simulink model "EISGov_SelectParameter"  (R2016b)
settings: configuration reference "CodeGenConfigSet" (kept outside this file)
values from neighbouring files (symbols this model uses):
  EISGov_SetPLoRmpSlopeNeg_C = Calibration.Parameter    [init_EISGov_SelectParameter.m]    (also in init_EISGov_SelectParameter_SIL.m = Simulink.Parameter)
  EISGov_SetPLoRmpSlopePos_C = Calibration.Parameter    [init_EISGov_SelectParameter.m]    (also in init_EISGov_SelectParameter_SIL.m = Simulink.Parameter)
  EISGov_stPrio_CA = Calibration.Parameter    [init_EISGov_SelectParameter.m]    (also in init_EISGov_SelectParameter_SIL.m = Simulink.Parameter)
undefined symbols (not defined in the file or in its folder): EISGov_num_conv, EISGov_SelectParameter_DT, Switch_conv
libraries: simulink x20, CXLib x3
(part 1 of 2)
settings Model: Creator=lenovo  LastModifiedBy=xuxingpei
settings ConfigSetRef: SourceLocation=Base Workspace

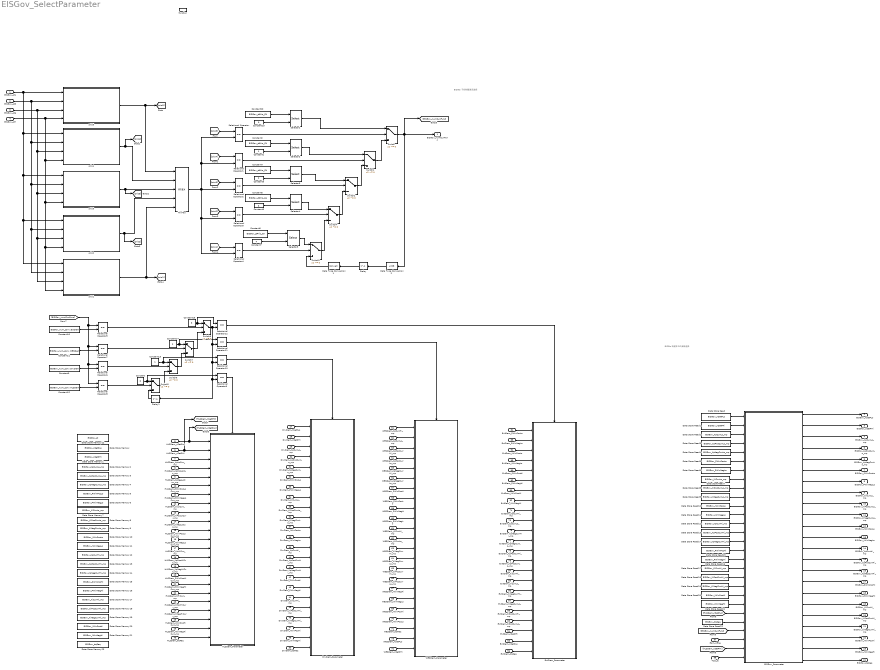
== system EISGov_SelectParameter ==
  note: EISGov转速和PID参数选择
  note: EISGov子控制器激活选择
  EISGov_st1 : Inport  Description=Status information of HLSDem client  OutMin=0  OutMax=2147483648  OutDataTypeStr=State_uint32
  EISGov_st3 : Inport  Description=Status information of WESDem client  Port=2  OutMin=0  OutMax=2147483648  OutDataTypeStr=State_uint32
  EISGov_st6 : Inport  Description=Status information of ExtDem client  Port=3  OutMin=0  OutMax=2147483648  OutDataTypeStr=State_uint32
  EISGov_st7 : Inport  Description=Status information of DrvDem client  Port=4  OutMin=0  OutMax=2147483648  OutDataTypeStr=State_uint32
  HLSDem_nSetPLo : Inport  Tag=rpm  Description=Minimum engine speed of HLSDem  Port=5  OutMin=0  OutMax=6000  OutDataTypeStr=EngSpeed_rpm
  HLSDem_nSetPHi : Inport  Tag=rpm  Description=Maximum engine speed of HLSDem  Port=6  OutMin=0  OutMax=6000  OutDataTypeStr=EngSpeed_rpm
  HLSDem_KpLoCurr_mp : Inport  Tag=Nm/rpm  Description=Current gain of the P-element of lower path  Port=7  OutMin=-10000  OutMax=10000  OutDataTypeStr=HLSDem_Kp
  HLSDem_KpPosLoCurr_mp : Inport  Tag=Nm/rpm  Description=Current positive large signal gain of the P-element of lower path  Port=8  OutMin=-10000  OutMax=10000  OutDataTypeStr=HLSDem_Kp
  HLSDem_KpNegLoCurr_mp : Inport  Tag=Nm/rpm  Description=Current negative large signal gain of the P-element of lower path  Port=9  OutMin=-10000  OutMax=10000  OutDataTypeStr=HLSDem_Kp
  HLSDem_PWinPosLoCurr_mp : Inport  Tag=rpm  Description=Current positive small-signal window P-component of the lower path  Port=10  OutMin=-6000  OutMax=6000  OutDataTypeStr=EngSpeed_rpm
  HLSDem_PWinNegLoCurr_mp : Inport  Tag=rpm  Description=Current negative small-signal window P-component of the lower path  Port=11  OutMin=-6000  OutMax=6000  OutDataTypeStr=EngSpeed_rpm
  HLSDem_KiLoCurr_mp : Inport  Tag=Nm/(rpm*s)  Description=Current gain of the I-element of lower path  Port=12  OutMin=-18000  OutMax=18000  OutDataTypeStr=HLSDem_Ki
  HLSDem_KiPosLoCurr_mp : Inport  Tag=Nm/(rpm*s)  Description=Current positive large signal gain of the I-element of lower path  Port=13  OutMin=-18000  OutMax=18000  OutDataTypeStr=HLSDem_Ki
  HLSDem_KiNegLoCurr_mp : Inport  Tag=Nm/(rpm*s)  Description=Current negative large signal gain of the I-element of lower path  Port=14  OutMin=-18000  OutMax=18000  OutDataTypeStr=HLSDem_Ki
  HLSDem_IWinPosLoCurr_mp : Inport  Tag=rpm  Description=Current positive small-signal window I-component of the lower path  Port=15  OutMin=-6000  OutMax=6000  OutDataTypeStr=EngSpeed_rpm
  HLSDem_IWinNegLoCurr_mp : Inport  Tag=rpm  Description=Current negative small-signal window I-component of the lower path  Port=16  OutMin=-6000  OutMax=6000  OutDataTypeStr=EngSpeed_rpm
  HLSDem_KpHiCurr_mp : Inport  Tag=Nm/rpm  Description=Current gain of the P-element of upper path  Port=17  OutMin=-10000  OutMax=10000  OutDataTypeStr=HLSDem_Kp
  HLSDem_KpPosHiCurr_mp : Inport  Tag=Nm/rpm  Description=Current positive large signal gain of the P-element of upper path  Port=18  OutMin=-10000  OutMax=10000  OutDataTypeStr=HLSDem_Kp
  HLSDem_KpNegHiCurr_mp : Inport  Tag=Nm/rpm  Description=Current negative large signal gain of the P-element of upper path  Port=19  OutMin=-10000  OutMax=10000  OutDataTypeStr=HLSDem_Kp
  HLSDem_PWinPosHiCurr_mp : Inport  Tag=rpm  Description=Current positive small-signal window P-component of the upper path  Port=20  OutMin=-6000  OutMax=6000  OutDataTypeStr=EngSpeed_rpm
  HLSDem_PWinNegHiCurr_mp : Inport  Tag=rpm  Description=Current negative small-signal window P-component of the upper path  Port=21  OutMin=-6000  OutMax=6000  OutDataTypeStr=EngSpeed_rpm
  HLSDem_KiHiCurr_mp : Inport  Tag=Nm/(rpm*s)  Description=Current small signal gain for the I component upper PI - path  Port=22  OutMin=-18000  OutMax=18000  OutDataTypeStr=HLSDem_Ki
  HLSDem_KiPosHiCurr_mp : Inport  Tag=Nm/(rpm*s)  Description=Current positive large signal gain for the I component upper PI-path  Port=23  OutMin=-18000  OutMax=18000  OutDataTypeStr=HLSDem_Ki
  HLSDem_KiNegHiCurr_mp : Inport  Tag=Nm/(rpm*s)  Description=Current negative large signal gain for the I component upper PI - path  Port=24  OutMin=-18000  OutMax=18000  OutDataTypeStr=HLSDem_Ki
  HLSDem_IWinPosHiCurr_mp : Inport  Tag=rpm  Description=Current positive small-signal window I-component of the upper path  Port=25  OutMin=-6000  OutMax=6000  OutDataTypeStr=EngSpeed_rpm
  HLSDem_IWinNegHiCurr_mp : Inport  Tag=rpm  Description=Current negative small-signal window I-component of the upper path  Port=26  OutMin=-6000  OutMax=6000  OutDataTypeStr=EngSpeed_rpm
  DrvDem_nSetPLo : Inport  Tag=rpm  Description=Minimal engine speed of DrvDem  Port=27  OutMin=0  OutMax=6000  OutDataTypeStr=EngSpeed_rpm
  DrvDem_nSetPHi : Inport  Tag=rpm  Description=Maximal engine speed of DrvDem  Port=28  OutMin=0  OutMax=6000  OutDataTypeStr=EngSpeed_rpm
  DrvDem_KpCurrLo_mp : Inport  Tag=Nm/rpm  Description=Current gain for the P element for the lower path  Port=29  OutMin=-10000  OutMax=10000  OutDataTypeStr=HLSDem_Kp
  DrvDem_KpPosCurrLo_mp : Inport  Tag=Nm/rpm  Description=Current positive large signal gain for the P component lower PI-path  Port=30  OutMin=-10000  OutMax=10000  OutDataTypeStr=HLSDem_Kp
  DrvDem_KpNegCurrLo_mp : Inport  Tag=Nm/rpm  Description=Current negative large signal gain for the P component lower PI-path  Port=31  OutMin=-10000  OutMax=10000  OutDataTypeStr=HLSDem_Kp
  DrvDem_PWinPosLo : Inport  Tag=rpm  Description=P component Positive window for parameterset lower PI- path  Port=32  OutMin=-6000  OutMax=6000  OutDataTypeStr=EngSpeed_rpm
  DrvDem_PWinNegLo : Inport  Tag=rpm  Description=P component negative window for parameterset lower PI- path  Port=33  OutMin=-6000  OutMax=6000  OutDataTypeStr=EngSpeed_rpm
  DrvDem_KiCurrLo_mp : Inport  Tag=Nm/(rpm*s)  Description=Current gain for the I element for the lower path  Port=34  OutMin=-18000  OutMax=18000  OutDataTypeStr=HLSDem_Ki
  DrvDem_KiPosCurrLo_mp : Inport  Tag=Nm/(rpm*s)  Description=Current positive large signal gain for the I component lower PI-path  Port=35  OutMin=-18000  OutMax=18000  OutDataTypeStr=HLSDem_Ki
  DrvDem_KiNegCurrLo_mp : Inport  Tag=Nm/(rpm*s)  Description=Current negative large signal gain for the I component lower PI-path  Port=36  OutMin=-18000  OutMax=18000  OutDataTypeStr=HLSDem_Ki
  DrvDem_IWinPosLo : Inport  Tag=rpm  Description=I component Positive window for parameterset lower PI- path  Port=37  OutMin=-6000  OutMax=6000  OutDataTypeStr=EngSpeed_rpm
  DrvDem_IWinNegLo : Inport  Tag=rpm  Description=I component negative window for parameterset lower PI- path  Port=38  OutMin=-6000  OutMax=6000  OutDataTypeStr=EngSpeed_rpm
  DrvDem_KpCurrHi_mp : Inport  Tag=Nm/rpm  Description=Current gain for the P element for the upper path  Port=39  OutMin=-10000  OutMax=10000  OutDataTypeStr=HLSDem_Kp
  DrvDem_KpPosCurrHi_mp : Inport  Tag=Nm/rpm  Description=Current positive large signal gain for the P component upper PI-path  Port=40  OutMin=-10000  OutMax=10000  OutDataTypeStr=HLSDem_Kp
  DrvDem_KpNegCurrHi_mp : Inport  Tag=Nm/rpm  Description=Current negative large signal gain for the P component upper PI-path  Port=41  OutMin=-10000  OutMax=10000  OutDataTypeStr=HLSDem_Kp
  DrvDem_PWinPosHi : Inport  Tag=rpm  Description=P component Positive window for parameterset upper PI- path  Port=42  OutMin=-6000  OutMax=6000  OutDataTypeStr=EngSpeed_rpm
  DrvDem_PWinNegHi : Inport  Tag=rpm  Description=P component negative window for parameterset upper PI- path  Port=43  OutMin=-6000  OutMax=6000  OutDataTypeStr=EngSpeed_rpm
  DrvDem_KiCurrHi_mp : Inport  Tag=Nm/(rpm*s)  Description=Current gain for the I element for the upper path  Port=44  OutMin=-18000  OutMax=18000  OutDataTypeStr=HLSDem_Ki
  DrvDem_KiPosCurrHi_mp : Inport  Tag=Nm/(rpm*s)  Description=Current positive large signal gain for the I component upper PI-path  Port=45  OutMin=-18000  OutMax=18000  OutDataTypeStr=HLSDem_Ki
  DrvDem_KiNegCurrHi_mp : Inport  Tag=Nm/(rpm*s)  Description=Current negative large signal gain for the I component upper PI-path  Port=46  OutMin=-18000  OutMax=18000  OutDataTypeStr=HLSDem_Ki
  DrvDem_IWinPosHi : Inport  Tag=rpm  Description=I component Positive window for parameterset upper PI- path  Port=47  OutMin=-6000  OutMax=6000  OutDataTypeStr=EngSpeed_rpm
  DrvDem_IWinNegHi : Inport  Tag=rpm  Description=I component negative window for parameterset upper PI- path  Port=48  OutMin=-6000  OutMax=6000  OutDataTypeStr=EngSpeed_rpm
  HLSDem_trqReq : Inport  Tag=Nm  Description=Requested initialisation torque to engine speed governor (with reference to the output)  Port=49  OutMin=-3000  OutMax=3000  OutDataTypeStr=Trq_Nm
  DrvDem_trqReq : Inport  Tag=Nm  Description=Requested initialisation torque to engine speed governor from DrvDem (with reference to the output)  Port=50  OutMin=-3000  OutMax=3000  OutDataTypeStr=Trq_Nm
  WESDem_KpCurrHi_mp : Inport  Tag=Nm/rpm  Description=Current small signal gain for the higher P component  Port=51  OutMin=-10000  OutMax=10000  OutDataTypeStr=HLSDem_Kp
  WESDem_KpCurrLo_mp : Inport  Tag=Nm/rpm  Description=Current small signal gain for the lower P component  Port=52  OutMin=-10000  OutMax=10000  OutDataTypeStr=HLSDem_Kp
  WESDem_KpPosCurrHi_mp : Inport  Tag=Nm/rpm  Description=Current positive large signal gain for the higher P component  Port=53  OutMin=-10000  OutMax=10000  OutDataTypeStr=HLSDem_Kp
  WESDem_KpPosCurrLo_mp : Inport  Tag=Nm/rpm  Description=Current positive large signal gain for the lower P component  Port=54  OutMin=-10000  OutMax=10000  OutDataTypeStr=HLSDem_Kp
  WESDem_KpNegCurrHi_mp : Inport  Tag=Nm/rpm  Description=Current negative large signal gain for the higher P component  Port=55  OutMin=-10000  OutMax=10000  OutDataTypeStr=HLSDem_Kp
  WESDem_KpNegCurrLo_mp : Inport  Tag=Nm/rpm  Description=Current negative large signal gain for the lower P component  Port=56  OutMin=-10000  OutMax=10000  OutDataTypeStr=HLSDem_Kp
  WESDem_PWinPosHi : Inport  Tag=rpm  Description=Positive higher small signal window for proportional component  Port=57  OutMin=-6000  OutMax=6000  OutDataTypeStr=EngSpeed_rpm
  WESDem_PWinPosLo : Inport  Tag=rpm  Description=Positive lower small signal window for proportional component  Port=58  OutMin=-6000  OutMax=6000  OutDataTypeStr=EngSpeed_rpm
  WESDem_PWinNegHi : Inport  Tag=rpm  Description=Negative higher small signal window for proportional component  Port=59  OutMin=-6000  OutMax=6000  OutDataTypeStr=EngSpeed_rpm
  WESDem_PWinNegLo : Inport  Tag=rpm  Description=Negative lower small signal window for proportional component  Port=60  OutMin=-6000  OutMax=6000  OutDataTypeStr=EngSpeed_rpm
  WESDem_KiCurrHi_mp : Inport  Tag=Nm/(rpm*s)  Description=Current small signal gain for the higher I component  Port=61  OutMin=-18000  OutMax=18000  OutDataTypeStr=HLSDem_Ki
  WESDem_KiCurrLo_mp : Inport  Tag=Nm/(rpm*s)  Description=Current small signal gain for the lower I component  Port=62  OutMin=-18000  OutMax=18000  OutDataTypeStr=HLSDem_Ki
  WESDem_KiNegCurrHi_mp : Inport  Tag=Nm/(rpm*s)  Description=Current negative large signal gain for the higher I component  Port=63  OutMin=-18000  OutMax=18000  OutDataTypeStr=HLSDem_Ki
  WESDem_KiNegCurrLo_mp : Inport  Tag=Nm/(rpm*s)  Description=Current negative large signal gain for the lower I component  Port=64  OutMin=-18000  OutMax=18000  OutDataTypeStr=HLSDem_Ki
  WESDem_KiPosCurrHi_mp : Inport  Tag=Nm/(rpm*s)  Description=Current positive large signal gain for the higher I component  Port=65  OutMin=-18000  OutMax=18000  OutDataTypeStr=HLSDem_Ki
  WESDem_KiPosCurrLo_mp : Inport  Tag=Nm/(rpm*s)  Description=Current positive large signal gain for the lower I component  Port=66  OutMin=-18000  OutMax=18000  OutDataTypeStr=HLSDem_Ki
  WESDem_IWinNegHi : Inport  Tag=rpm  Description=Negative higher small signal window for integral component  Port=67  OutMin=-6000  OutMax=6000  OutDataTypeStr=EngSpeed_rpm
  WESDem_IWinNegLo : Inport  Tag=rpm  Description=Negative lower small signal window for integral component  Port=68  OutMin=-6000  OutMax=6000  OutDataTypeStr=EngSpeed_rpm
  WESDem_IWinPosHi : Inport  Tag=rpm  Description=Positive higher small signal window for integral component  Port=69  OutMin=-6000  OutMax=6000  OutDataTypeStr=EngSpeed_rpm
  WESDem_IWinPosLo : Inport  Tag=rpm  Description=Positive lower small signal window for integral component  Port=70  OutMin=-6000  OutMax=6000  OutDataTypeStr=EngSpeed_rpm
  WESDem_trqReq : Inport  Tag=Nm  Description=Torque intialization request of working engine speed demand  Port=71  OutMin=-3276  OutMax=3276  OutDataTypeStr=Trq_Nm
  WESDem_nSetPHi : Inport  Tag=rpm  Description=Higher setpoint speed interval of WESDem  Port=72  OutMin=0  OutMax=6000  OutDataTypeStr=EngSpeed_rpm
  WESDem_nSetPLo : Inport  Tag=rpm  Description=Lower setpoint speed interval of WESDem  Port=73  OutMin=0  OutMax=6000  OutDataTypeStr=EngSpeed_rpm
  ExtDem_KpCurrHi_mp : Inport  Tag=Nm/rpm  Description=Current small signal gain for the P higher component  Port=74  OutMin=-10000  OutMax=10000  OutDataTypeStr=HLSDem_Kp
  ExtDem_KpCurrLo_mp : Inport  Tag=Nm/rpm  Description=Current small signal gain for the P lower component  Port=75  OutMin=-10000  OutMax=10000  OutDataTypeStr=HLSDem_Kp
  ExtDem_KpNegCurrHi_mp : Inport  Tag=Nm/rpm  Description=Current negative large signal gain for the P higher component  Port=76  OutMin=-10000  OutMax=10000  OutDataTypeStr=HLSDem_Kp
  ExtDem_KpNegCurrLo_mp : Inport  Tag=Nm/rpm  Description=Current negative large signal gain for the lower P component  Port=77  OutMin=-10000  OutMax=10000  OutDataTypeStr=HLSDem_Kp
  ExtDem_KpPosCurrHi_mp : Inport  Tag=Nm/rpm  Description=Current positive large signal gain for the P higher component  Port=78  OutMin=-10000  OutMax=10000  OutDataTypeStr=HLSDem_Kp
  ExtDem_KpPosCurrLo_mp : Inport  Tag=Nm/rpm  Description=Current positive large signal gain for the P lower component  Port=79  OutMin=-10000  OutMax=10000  OutDataTypeStr=HLSDem_Kp
  ExtDem_PWinPosHi : Inport  Tag=rpm  Description=Positive small signal window for proportional higher component  Port=80  OutMin=-1000  OutMax=1000  OutDataTypeStr=EngSpeed_rpm
  ExtDem_PWinPosLo : Inport  Tag=rpm  Description=Positive small signal window for proportional lower component  Port=81  OutMin=-1000  OutMax=1000  OutDataTypeStr=EngSpeed_rpm
  ExtDem_PWinNegHi : Inport  Tag=rpm  Description=Negative small signal window for proportional higher component  Port=82  OutMin=-1000  OutMax=1000  OutDataTypeStr=EngSpeed_rpm
  ExtDem_PWinNegLo : Inport  Tag=rpm  Description=Negative small signal window for proportional lower component  Port=83  OutMin=-1000  OutMax=1000  OutDataTypeStr=EngSpeed_rpm
  ExtDem_KiCurrHi_mp : Inport  Tag=Nm/(rpm*s)  Description=Current small signal gain for the I higher component  Port=84  OutMin=-18000  OutMax=18000  OutDataTypeStr=HLSDem_Ki
  ExtDem_KiCurrLo_mp : Inport  Tag=Nm/(rpm*s)  Description=Current small signal gain for the I lower component  Port=85  OutMin=-18000  OutMax=18000  OutDataTypeStr=HLSDem_Ki
  ExtDem_KiNegCurrHi_mp : Inport  Tag=Nm/(rpm*s)  Description=Current negative large signal gain for the I higher component  Port=86  OutMin=-18000  OutMax=18000  OutDataTypeStr=HLSDem_Ki
  ExtDem_KiNegCurrLo_mp : Inport  Tag=Nm/(rpm*s)  Description=Current negative large signal gain for the I lower component  Port=87  OutMin=-18000  OutMax=18000  OutDataTypeStr=HLSDem_Ki
  ExtDem_KiPosCurrHi_mp : Inport  Tag=Nm/(rpm*s)  Description=Current positive large signal gain for the I higher component  Port=88  OutMin=-18000  OutMax=18000  OutDataTypeStr=HLSDem_Ki
  ExtDem_KiPosCurrLo_mp : Inport  Tag=Nm/(rpm*s)  Description=Current positive large signal gain for the I lower component  Port=89  OutMin=-18000  OutMax=18000  OutDataTypeStr=HLSDem_Ki
  ExtDem_IWinPosHi : Inport  Tag=rpm  Description=Positive small signal window for integral higher component  Port=90  OutMin=-1000  OutMax=1000  OutDataTypeStr=EngSpeed_rpm
  ExtDem_IWinPosLo : Inport  Tag=rpm  Description=Positive small signal window for integral lower component  Port=91  OutMin=-1000  OutMax=1000  OutDataTypeStr=EngSpeed_rpm
  ExtDem_IWinNegHi : Inport  Tag=rpm  Description=Negative small signal window for integral higher component  Port=92  OutMin=-1000  OutMax=1000  OutDataTypeStr=EngSpeed_rpm
  ExtDem_IWinNegLo : Inport  Tag=rpm  Description=Negative small signal window for integral lower component  Port=93  OutMin=-1000  OutMax=1000  OutDataTypeStr=EngSpeed_rpm
  ExtDem_nSetPHi : Inport  Tag=rpm  Description=Higher limit of external demand set point speed  Port=94  OutMin=0  OutMax=6000  OutDataTypeStr=EngSpeed_rpm
  ExtDem_nSetPLo : Inport  Tag=rpm  Description=Lower limit of external demand set point speed  Port=95  OutMin=0  OutMax=6000  OutDataTypeStr=EngSpeed_rpm
  ExtDem_trqReq : Inport  Tag=Nm  Description=|  Port=96  OutMin=-3000  OutMax=3000  OutDataTypeStr=Trq_Nm
      | Torque intialization request of the EISGov External
      | Intervention function
  Epm_nEng : Inport  Tag=rpm  Description=Engine speed  Port=97  OutMin=0  OutMax=6000  OutDataTypeStr=EngSpeed_rpm
  T15_st : Inport  Description=Terminal 15 status after debouncing  Port=98  OutDataTypeStr=Enum: Switch_conv
  function : TriggerPort  TriggerType=function-call  VariantControl=Variant
  Constant : Constant  Value=0  OutDataTypeStr=Inherit: Inherit via back propagation
  Constant1 : Constant  OutDataTypeStr=uint8
  Constant10 : Constant  Value=EISGov_num_conv.ExtDem
  Constant11 : Constant  Value=EISGov_num_conv.WESDem
  Constant12 : Constant  Value=EISGov_num_conv.HLSDem
  Constant13 : Constant  OutDataTypeStr=Inherit: Inherit via back propagation
  Constant14 : Constant  Value=2  OutDataTypeStr=Inherit: Inherit via back propagation
  Constant15 : Constant  Value=0  OutDataTypeStr=uint8
  Constant16 : Constant  Value=3  OutDataTypeStr=uint8
  Constant{2,4,6,8,20} (5 alike) : Constant  Value=EISGov_stPrio_CA
  Constant3 : Constant  Value=2  OutDataTypeStr=uint8
  Constant5 : Constant  Value=3  OutDataTypeStr=uint8
  Constant7 : Constant  Value=4  OutDataTypeStr=uint8
  Constant9 : Constant  Value=EISGov_num_conv.DrvDem
  Data Store Memory : DataStoreMemory  DataStoreName=EISGov_nSetPLo  ReadBeforeWriteMsg=warning  WriteAfterWriteMsg=warning  WriteAfterReadMsg=warning  ShowAdditionalParam=off
  Data Store Memory1 : DataStoreMemory  DataStoreName=EISGov_nSetPHi  ReadBeforeWriteMsg=warning  WriteAfterWriteMsg=warning  WriteAfterReadMsg=warning  ShowAdditionalParam=off
  Data Store Memory10 : DataStoreMemory  DataStoreName=EISGov_IWinPosLo  ReadBeforeWriteMsg=warning  WriteAfterWriteMsg=warning  WriteAfterReadMsg=warning  ShowAdditionalParam=off
  Data Store Memory11 : DataStoreMemory  DataStoreName=EISGov_IWinNegLo  ReadBeforeWriteMsg=warning  WriteAfterWriteMsg=warning  WriteAfterReadMsg=warning  ShowAdditionalParam=off
  Data Store Memory12 : DataStoreMemory  DataStoreName=EISGov_KpCurrHi_mp  ReadBeforeWriteMsg=warning  WriteAfterWriteMsg=warning  WriteAfterReadMsg=warning  ShowAdditionalParam=off
  Data Store Memory13 : DataStoreMemory  DataStoreName=EISGov_KpPosCurrHi_mp  ReadBeforeWriteMsg=warning  WriteAfterWriteMsg=warning  WriteAfterReadMsg=warning  ShowAdditionalParam=off
  Data Store Memory14 : DataStoreMemory  DataStoreName=EISGov_KpNegCurrHi_mp  ReadBeforeWriteMsg=warning  WriteAfterWriteMsg=warning  WriteAfterReadMsg=warning  ShowAdditionalParam=off
  Data Store Memory15 : DataStoreMemory  DataStoreName=EISGov_PWinPosHi  ReadBeforeWriteMsg=warning  WriteAfterWriteMsg=warning  WriteAfterReadMsg=warning  ShowAdditionalParam=off
  Data Store Memory16 : DataStoreMemory  DataStoreName=EISGov_PWinNegHi  ReadBeforeWriteMsg=warning  WriteAfterWriteMsg=warning  WriteAfterReadMsg=warning  ShowAdditionalParam=off
  Data Store Memory17 : DataStoreMemory  DataStoreName=EISGov_KiCurrHi_mp  ReadBeforeWriteMsg=warning  WriteAfterWriteMsg=warning  WriteAfterReadMsg=warning  ShowAdditionalParam=off
  Data Store Memory18 : DataStoreMemory  DataStoreName=EISGov_KiPosCurrHi_mp  ReadBeforeWriteMsg=warning  WriteAfterWriteMsg=warning  WriteAfterReadMsg=warning  ShowAdditionalParam=off
  Data Store Memory19 : DataStoreMemory  DataStoreName=EISGov_KiNegCurrHi_mp  ReadBeforeWriteMsg=warning  WriteAfterWriteMsg=warning  WriteAfterReadMsg=warning  ShowAdditionalParam=off
  Data Store Memory2 : DataStoreMemory  DataStoreName=EISGov_KpCurrLo_mp  ReadBeforeWriteMsg=warning  WriteAfterWriteMsg=warning  WriteAfterReadMsg=warning  ShowAdditionalParam=off
  Data Store Memory20 : DataStoreMemory  DataStoreName=EISGov_IWinPosHi  ReadBeforeWriteMsg=warning  WriteAfterWriteMsg=warning  WriteAfterReadMsg=warning  ShowAdditionalParam=off
  Data Store Memory21 : DataStoreMemory  DataStoreName=EISGov_IWinNegHi  ReadBeforeWriteMsg=warning  WriteAfterWriteMsg=warning  WriteAfterReadMsg=warning  ShowAdditionalParam=off
  Data Store Memory22 : DataStoreMemory  DataStoreName=EISGov_st  ReadBeforeWriteMsg=warning  WriteAfterWriteMsg=warning  WriteAfterReadMsg=warning  ShowAdditionalParam=off
  Data Store Memory23 : DataStoreMemory  DataStoreName=EISGov_trqReq  ReadBeforeWriteMsg=warning  WriteAfterWriteMsg=warning  WriteAfterReadMsg=warning  ShowAdditionalParam=off
  Data Store Memory3 : DataStoreMemory  DataStoreName=EISGov_KpPosCurrLo_mp  ReadBeforeWriteMsg=warning  WriteAfterWriteMsg=warning  WriteAfterReadMsg=warning  ShowAdditionalParam=off
  Data Store Memory4 : DataStoreMemory  DataStoreName=EISGov_KpNegCurrLo_mp  ReadBeforeWriteMsg=warning  WriteAfterWriteMsg=warning  WriteAfterReadMsg=warning  ShowAdditionalParam=off
  Data Store Memory5 : DataStoreMemory  DataStoreName=EISGov_PWinPosLo  ReadBeforeWriteMsg=warning  WriteAfterWriteMsg=warning  WriteAfterReadMsg=warning  ShowAdditionalParam=off
  Data Store Memory6 : DataStoreMemory  DataStoreName=EISGov_PWinNegLo  ReadBeforeWriteMsg=warning  WriteAfterWriteMsg=warning  WriteAfterReadMsg=warning  ShowAdditionalParam=off
  Data Store Memory7 : DataStoreMemory  DataStoreName=EISGov_KiCurrLo_mp  ReadBeforeWriteMsg=warning  WriteAfterWriteMsg=warning  WriteAfterReadMsg=warning  ShowAdditionalParam=off
  Data Store Memory8 : DataStoreMemory  DataStoreName=EISGov_KiPosCurrLo_mp  ReadBeforeWriteMsg=warning  WriteAfterWriteMsg=warning  WriteAfterReadMsg=warning  ShowAdditionalParam=off
  Data Store Memory9 : DataStoreMemory  DataStoreName=EISGov_KiNegCurrLo_mp  ReadBeforeWriteMsg=warning  WriteAfterWriteMsg=warning  WriteAfterReadMsg=warning  ShowAdditionalParam=off
  Data Store Read : DataStoreRead  DataStoreName=EISGov_nSetPLo
  Data Store Read1 : DataStoreRead  DataStoreName=EISGov_nSetPHi
  Data Store Read10 : DataStoreRead  DataStoreName=EISGov_IWinPosLo
  Data Store Read11 : DataStoreRead  DataStoreName=EISGov_IWinNegLo
  Data Store Read12 : DataStoreRead  DataStoreName=EISGov_KpCurrHi_mp
  Data Store Read13 : DataStoreRead  DataStoreName=EISGov_KpPosCurrHi_mp
  Data Store Read14 : DataStoreRead  DataStoreName=EISGov_KpNegCurrHi_mp
  Data Store Read15 : DataStoreRead  DataStoreName=EISGov_PWinPosHi
  Data Store Read16 : DataStoreRead  DataStoreName=EISGov_PWinNegHi
  Data Store Read17 : DataStoreRead  DataStoreName=EISGov_KiCurrHi_mp
  Data Store Read18 : DataStoreRead  DataStoreName=EISGov_KiPosCurrHi_mp
  Data Store Read19 : DataStoreRead  DataStoreName=EISGov_KiNegCurrHi_mp
  Data Store Read2 : DataStoreRead  DataStoreName=EISGov_KpCurrLo_mp
  Data Store Read20 : DataStoreRead  DataStoreName=EISGov_IWinPosHi
  Data Store Read21 : DataStoreRead  DataStoreName=EISGov_IWinNegHi
  Data Store Read22 : DataStoreRead  DataStoreName=EISGov_trqReq
  Data Store Read3 : DataStoreRead  DataStoreName=EISGov_KpPosCurrLo_mp
  Data Store Read4 : DataStoreRead  DataStoreName=EISGov_KpNegCurrLo_mp
  Data Store Read5 : DataStoreRead  DataStoreName=EISGov_PWinPosLo
  Data Store Read6 : DataStoreRead  DataStoreName=EISGov_PWinNegLo
  Data Store Read7 : DataStoreRead  DataStoreName=EISGov_KiCurrLo_mp
  Data Store Read8 : DataStoreRead  DataStoreName=EISGov_KiPosCurrLo_mp
  Data Store Read9 : DataStoreRead  DataStoreName=EISGov_KiNegCurrLo_mp
  Data Type Conversion1 : DataTypeConversion
  Data Type Conversion2 : DataTypeConversion  OutDataTypeStr=uint8
  Delay : Delay  DelayLength=1  InitialCondition=0
  Delay1 : Delay  DelayLength=1  InitialCondition=0
  DrvDem_Parameter : Subsystem  TreatAsAtomicUnit=on
  EISGov_Parameter : Subsystem
  ExtDem_Parameter : Subsystem  TreatAsAtomicUnit=on
  HLSDem_Parameter : Subsystem  TreatAsAtomicUnit=on
  MinMax : MinMax  Function=max  Inputs=5
  Relational Operator{,1..12} (13 alike) : RelationalOperator  Operator===  OutDataTypeStr=boolean  RndMeth=Simplest
  Selector{1..5} (5 alike) : Selector  IndexMode=Zero-based  IndexOptions=Index vector (port)  Indices=[1 3]  OutputSizes=1
  Switch{,1..8} (9 alike) : Switch  Criteria=u2 ~= 0
  WESDem_Parameter : Subsystem  TreatAsAtomicUnit=on
  prio1 : Subsystem
  prio2 : Subsystem
  prio3 : Subsystem
  prio4 : Subsystem
  prio5 : Subsystem
  EISGov_numCurrFunc : Outport  Description=Identification name / number of the currently active EISGov client, which determines the current controller parameters  OutDataTypeStr=Enum: EISGov_num_conv
  EISGov_nSetPLo : Outport  Tag=rpm  Description=Lower limit of the speed interval (set point speed) of the EISGov  Port=2  OutMin=0  OutMax=6000  OutDataTypeStr=EngSpeed_rpm
  EISGov_nSetPHi : Outport  Tag=rpm  Description=Upper limit of the speed interval (maximum speed) of EISGov  Port=3  OutMin=0  OutMax=6000  OutDataTypeStr=EngSpeed_rpm
  EISGov_KpCurrLo_mp : Outport  Tag=Nm/rpm  Description=Current gain for the P element for the lower path  Port=4  OutMin=-10000  OutMax=10000  OutDataTypeStr=HLSDem_Kp
  EISGov_KpPosCurrLo_mp : Outport  Tag=Nm/rpm  Description=Current positive large signal gain for the P component lower PI-path  Port=5  OutMin=-10000  OutMax=10000  OutDataTypeStr=HLSDem_Kp
  EISGov_KpNegCurrLo_mp : Outport  Tag=Nm/rpm  Description=Current negative large signal gain for the P component lower PI-path  Port=6  OutMin=-10000  OutMax=10000  OutDataTypeStr=HLSDem_Kp
  EISGov_PWinPosLo : Outport  Tag=rpm  Description=P component Positive window for parameterset lower PI- path  Port=7  OutMin=-6000  OutMax=6000  OutDataTypeStr=EngSpeed_rpm
  EISGov_PWinNegLo : Outport  Tag=rpm  Description=P component negative window for parameterset lower PI- path  Port=8  OutMin=-6000  OutMax=6000  OutDataTypeStr=EngSpeed_rpm
  EISGov_KiCurrLo_mp : Outport  Tag=Nm/(rpm*s)  Description=Current gain for the I element for the lower path  Port=9  OutMin=-18000  OutMax=18000  OutDataTypeStr=HLSDem_Ki
  EISGov_KiPosCurrLo_mp : Outport  Tag=Nm/(rpm*s)  Description=Current positive large signal gain for the I component lower PI-path  Port=10  OutMin=-18000  OutMax=18000  OutDataTypeStr=HLSDem_Ki
  EISGov_KiNegCurrLo_mp : Outport  Tag=Nm/(rpm*s)  Description=Current negative large signal gain for the I component lower PI-path  Port=11  OutMin=-18000  OutMax=18000  OutDataTypeStr=HLSDem_Ki
  EISGov_IWinPosLo : Outport  Tag=rpm  Description=I component Positive window for parameterset lower PI- path  Port=12  OutMin=-6000  OutMax=6000  OutDataTypeStr=EngSpeed_rpm
  EISGov_IWinNegLo : Outport  Tag=rpm  Description=I component negative window for parameterset lower PI- path  Port=13  OutMin=-6000  OutMax=6000  OutDataTypeStr=EngSpeed_rpm
  EISGov_KpCurrHi_mp : Outport  Tag=Nm/rpm  Description=Current gain for the P element for the upper path  Port=14  OutMin=-10000  OutMax=10000  OutDataTypeStr=HLSDem_Kp
  EISGov_KpPosCurrHi_mp : Outport  Tag=Nm/rpm  Description=Current positive large signal gain for the P component upper PI-path  Port=15  OutMin=-10000  OutMax=10000  OutDataTypeStr=HLSDem_Kp
  EISGov_KpNegCurrHi_mp : Outport  Tag=Nm/rpm  Description=Current negative large signal gain for the P component upper PI-path  Port=16  OutMin=-10000  OutMax=10000  OutDataTypeStr=HLSDem_Kp
  EISGov_PWinPosHi : Outport  Tag=rpm  Description=P component Positive window for parameterset upper PI- path  Port=17  OutMin=-6000  OutMax=6000  OutDataTypeStr=EngSpeed_rpm
  EISGov_PWinNegHi : Outport  Tag=rpm  Description=P component negative window for parameterset upper PI- path  Port=18  OutMin=-6000  OutMax=6000  OutDataTypeStr=EngSpeed_rpm
  EISGov_KiCurrHi_mp : Outport  Tag=Nm/(rpm*s)  Description=Current gain for the I element for the upper path  Port=19  OutMin=-18000  OutMax=18000  OutDataTypeStr=HLSDem_Ki
  EISGov_KiPosCurrHi_mp : Outport  Tag=Nm/(rpm*s)  Description=Current positive large signal gain for the I component upper PI-path  Port=20  OutMin=-18000  OutMax=18000  OutDataTypeStr=HLSDem_Ki
  EISGov_KiNegCurrHi_mp : Outport  Tag=Nm/(rpm*s)  Description=Current negative large signal gain for the I component upper PI-path  Port=21  OutMin=-18000  OutMax=18000  OutDataTypeStr=HLSDem_Ki
  EISGov_IWinPosHi : Outport  Tag=rpm  Description=I component Positive window for parameterset upper PI- path  Port=22  OutMin=-6000  OutMax=6000  OutDataTypeStr=EngSpeed_rpm
  EISGov_IWinNegHi : Outport  Tag=rpm  Description=I component negative window for parameterset upper PI- path  Port=23  OutMin=-6000  OutMax=6000  OutDataTypeStr=EngSpeed_rpm
  EISGov_trqReq : Outport  Tag=Nm  Description=Selected requirement (from all the requirements of the active EISGov clients) to the EISGov for an initialisation torque  Port=24  OutMin=-3276.8  OutMax=3276.7  OutDataTypeStr=Trq_Nm
  wires:
  prio5/1(prio5) -> [prio5], MinMax/1
  prio1/1(prio1) -> [prio1], MinMax/5
  [prio5] -> Relational Operator/1
  [prio4] -> Relational Operator1/1
  prio4/1(prio4) -> [prio4], MinMax/2
  prio2/1(prio2) -> [prio2], MinMax/4
  MinMax/1 -> Relational Operator4/2, Relational Operator3/2, Relational Operator1/2, Relational Operator/2, Relational Operator2/2
  [prio3] -> Relational Operator2/1
  [prio1] -> Relational Operator4/1
  Constant20/1 -> Selector1/1
  [prio2] -> Relational Operator3/1
  prio3/1(prio3) -> [prio3], MinMax/3
  Switch/1 -> EISGov_numCurrFunc/1, [EISGov_numCurrFunc], Data Type Conversion2/1  "EISGov_numCurrFunc"
  Constant3/1 -> Selector3/2
  Switch1/1 -> Switch/3
  Delay/1 -> Data Type Conversion1/1
  Constant6/1 -> Selector4/1
  Constant7/1 -> Selector5/2
  Constant15/1 -> Selector1/2
  Constant5/1 -> Selector4/2
  Switch4/1 -> Switch2/3
  Selector5/1 -> Switch3/1
  Constant4/1 -> Selector3/1
  Relational Operator3/1 -> Switch4/2
  Data Type Conversion1/1 -> Switch3/3
  Relational Operator/1 -> Switch/2
  Data Type Conversion2/1 -> Delay/1
  Data Store Read/1 -> EISGov_Parameter/1(EISGov_nSetPLo_IN)
  Relational Operator2/1 -> Switch2/2
  Data Store Read2/1 -> EISGov_Parameter/3(EISGov_KpCurrLo_mp_IN)
  Constant2/1 -> Selector2/1
  Data Store Read1/1 -> EISGov_Parameter/2(EISGov_nSetPHi_IN)
  Constant8/1 -> Selector5/1
  Data Store Read3/1 -> EISGov_Parameter/4(EISGov_KpPosCurrLo_mp_IN)
  Data Store Read4/1 -> EISGov_Parameter/5(EISGov_KpNegCurrLo_mp_IN)
  Switch2/1 -> Switch1/3
  Selector1/1 -> Switch/1
  Relational Operator1/1 -> Switch1/2
  Selector3/1 -> Switch2/1
  Relational Operator4/1 -> Switch3/2
  Switch3/1 -> Switch4/3
  Constant1/1 -> Selector2/2
  Selector4/1 -> Switch4/1
  Selector2/1 -> Switch1/1
  Data Store Read13/1 -> EISGov_Parameter/14(EISGov_KpPosCurrHi_mp_IN)
  Data Store Read21/1 -> EISGov_Parameter/22(EISGov_IWinNegHi_IN)
  [EISGov_numCurrFunc] -> Relational Operator5/1, Relational Operator6/1, Relational Operator8/1, Relational Operator7/1
  Data Store Read5/1 -> EISGov_Parameter/6(EISGov_PWinPosLo_IN)
  Constant10/1 -> Relational Operator5/2
  Data Store Read11/1 -> EISGov_Parameter/12(EISGov_IWinNegLo_IN)
  Data Store Read22/1 -> EISGov_Parameter/24(EISGov_trqReq_IN)
  Data Store Read8/1 -> EISGov_Parameter/9(EISGov_KiPosCurrLo_mp_IN)
  Data Store Read19/1 -> EISGov_Parameter/20(EISGov_KiNegCurrHi_mp_IN)
  Data Store Read10/1 -> EISGov_Parameter/11(EISGov_IWinPosLo_IN)
  Data Store Read7/1 -> EISGov_Parameter/8(EISGov_KiCurrLo_mp_IN)
  Data Store Read9/1 -> EISGov_Parameter/10(EISGov_KiNegCurrLo_mp_IN)
  Data Store Read12/1 -> EISGov_Parameter/13(EISGov_KpCurrHi_mp_IN)
  Data Store Read16/1 -> EISGov_Parameter/17(EISGov_PWinNegHi_IN)
  [HLSDem_nSetPLo] -> EISGov_Parameter/23(HLSDem_nSetPLo_IN)
  Constant12/1 -> Relational Operator8/2
  Data Store Read6/1 -> EISGov_Parameter/7(EISGov_PWinNegLo_IN)
  Data Store Read18/1 -> EISGov_Parameter/19(EISGov_KiPosCurrHi_mp_IN)
  Data Store Read17/1 -> EISGov_Parameter/18(EISGov_KiCurrHi_mp_IN)
  Constant9/1 -> Relational Operator6/2
  Constant11/1 -> Relational Operator7/2
  Data Store Read14/1 -> EISGov_Parameter/15(EISGov_KpNegCurrHi_mp_IN)
  Data Store Read20/1 -> EISGov_Parameter/21(EISGov_IWinPosHi_IN)
  Data Store Read15/1 -> EISGov_Parameter/16(EISGov_PWinPosHi_IN)
  [EISGov_numCurrFunc] -> EISGov_Parameter/25(EISGov_numCurrFunc)
  EISGov_Parameter/1(EISGov_nSetPLo) -> EISGov_nSetPLo/1  "EISGov_nSetPLo"
  EISGov_Parameter/2(EISGov_nSetPHi) -> EISGov_nSetPHi/1  "EISGov_nSetPHi"
  EISGov_Parameter/3(EISGov_KpCurrLo_mp) -> EISGov_KpCurrLo_mp/1  "EISGov_KpCurrLo_mp"
  EISGov_Parameter/4(EISGov_KpPosCurrLo_mp) -> EISGov_KpPosCurrLo_mp/1  "EISGov_KpPosCurrLo_mp"
  EISGov_Parameter/5(EISGov_KpNegCurrLo_mp) -> EISGov_KpNegCurrLo_mp/1  "EISGov_KpNegCurrLo_mp"
  EISGov_Parameter/6(EISGov_PWinPosLo) -> EISGov_PWinPosLo/1  "EISGov_PWinPosLo"
  EISGov_Parameter/7(EISGov_PWinNegLo) -> EISGov_PWinNegLo/1  "EISGov_PWinNegLo"
  EISGov_Parameter/8(EISGov_KiCurrLo_mp) -> EISGov_KiCurrLo_mp/1  "EISGov_KiCurrLo_mp"
  EISGov_Parameter/9(EISGov_KiPosCurrLo_mp) -> EISGov_KiPosCurrLo_mp/1  "EISGov_KiPosCurrLo_mp"
  EISGov_Parameter/10(EISGov_KiNegCurrLo_mp) -> EISGov_KiNegCurrLo_mp/1  "EISGov_KiNegCurrLo_mp"
  EISGov_Parameter/11(EISGov_IWinPosLo) -> EISGov_IWinPosLo/1  "EISGov_IWinPosLo"
  EISGov_Parameter/12(EISGov_IWinNegLo) -> EISGov_IWinNegLo/1  "EISGov_IWinNegLo"
  EISGov_Parameter/13(EISGov_KpCurrHi_mp) -> EISGov_KpCurrHi_mp/1  "EISGov_KpCurrHi_mp"
  EISGov_Parameter/14(EISGov_KpPosCurrHi_mp) -> EISGov_KpPosCurrHi_mp/1  "EISGov_KpPosCurrHi_mp"
  EISGov_Parameter/15(EISGov_KpNegCurrHi_mp) -> EISGov_KpNegCurrHi_mp/1  "EISGov_KpNegCurrHi_mp"
  EISGov_Parameter/16(EISGov_PWinPosHi) -> EISGov_PWinPosHi/1  "EISGov_PWinPosHi"
  EISGov_Parameter/17(EISGov_PWinNegHi) -> EISGov_PWinNegHi/1  "EISGov_PWinNegHi"
  EISGov_Parameter/18(EISGov_KiCurrHi_mp) -> EISGov_KiCurrHi_mp/1  "EISGov_KiCurrHi_mp"
  EISGov_Parameter/19(EISGov_KiPosCurrHi_mp) -> EISGov_KiPosCurrHi_mp/1  "EISGov_KiPosCurrHi_mp"
  EISGov_Parameter/20(EISGov_KiNegCurrHi_mp) -> EISGov_KiNegCurrHi_mp/1  "EISGov_KiNegCurrHi_mp"
  EISGov_Parameter/21(EISGov_IWinPosHi) -> EISGov_IWinPosHi/1  "EISGov_IWinPosHi"
  EISGov_Parameter/22(EISGov_IWinNegHi) -> EISGov_IWinNegHi/1  "EISGov_IWinNegHi"
  EISGov_Parameter/23(EISGov_trqReq) -> EISGov_trqReq/1  "EISGov_trqReq"
  HLSDem_nSetPHi/1 -> [HLSDem_nSetPHi], HLSDem_Parameter/2(HLSDem_nSetPHi)
  HLSDem_KiLoCurr_mp/1 -> HLSDem_Parameter/8(HLSDem_KiLoCurr_mp)
  HLSDem_PWinPosLoCurr_mp/1 -> HLSDem_Parameter/6(HLSDem_PWinPosLoCurr_mp)
  HLSDem_PWinNegHiCurr_mp/1 -> HLSDem_Parameter/17(HLSDem_PWinNegHiCurr_mp)
  HLSDem_KiHiCurr_mp/1 -> HLSDem_Parameter/18(HLSDem_KiHiCurr_mp)
  HLSDem_IWinNegHiCurr_mp/1 -> HLSDem_Parameter/22(HLSDem_IWinNegHiCurr_mp)
  HLSDem_KpLoCurr_mp/1 -> HLSDem_Parameter/3(HLSDem_KpLoCurr_mp)
  HLSDem_IWinNegLoCurr_mp/1 -> HLSDem_Parameter/12(HLSDem_IWinNegLoCurr_mp)
  HLSDem_KpNegLoCurr_mp/1 -> HLSDem_Parameter/5(HLSDem_KpNegLoCurr_mp)
  HLSDem_KiNegHiCurr_mp/1 -> HLSDem_Parameter/20(HLSDem_KiNegHiCurr_mp)
  HLSDem_KpPosHiCurr_mp/1 -> HLSDem_Parameter/14(HLSDem_KpPosHiCurr_mp)
  HLSDem_KiPosLoCurr_mp/1 -> HLSDem_Parameter/9(HLSDem_KiPosLoCurr_mp)
  HLSDem_PWinNegLoCurr_mp/1 -> HLSDem_Parameter/7(HLSDem_PWinNegLoCurr_mp)
  HLSDem_KiPosHiCurr_mp/1 -> HLSDem_Parameter/19(HLSDem_KiPosHiCurr_mp)
  HLSDem_KpNegHiCurr_mp/1 -> HLSDem_Parameter/15(HLSDem_KpNegHiCurr_mp)
  HLSDem_KpPosLoCurr_mp/1 -> HLSDem_Parameter/4(HLSDem_KpPosLoCurr_mp)
  HLSDem_KiNegLoCurr_mp/1 -> HLSDem_Parameter/10(HLSDem_KiNegLoCurr_mp)
  HLSDem_IWinPosHiCurr_mp/1 -> HLSDem_Parameter/21(HLSDem_IWinPosHiCurr_mp)
  HLSDem_KpHiCurr_mp/1 -> HLSDem_Parameter/13(HLSDem_KpHiCurr_mp)
  HLSDem_PWinPosHiCurr_mp/1 -> HLSDem_Parameter/16(HLSDem_PWinPosHiCurr_mp)
  HLSDem_trqReq/1 -> HLSDem_Parameter/23(HLSDem_trqReq)
  HLSDem_IWinPosLoCurr_mp/1 -> HLSDem_Parameter/11(HLSDem_IWinPosLoCurr_mp)
  HLSDem_nSetPLo/1 -> [HLSDem_nSetPLo], HLSDem_Parameter/1(HLSDem_nSetPLo)
  EISGov_st3/1 -> prio1/2(EISGov_st3), prio2/2(EISGov_st3), prio3/2(EISGov_st3), prio4/2(EISGov_st3), prio5/2(EISGov_st3)
  EISGov_st6/1 -> prio1/3(EISGov_st6), prio2/3(EISGov_st6), prio3/3(EISGov_st6), prio4/3(EISGov_st6), prio5/3(EISGov_st6)
  EISGov_st7/1 -> prio1/4(EISGov_st7), prio2/4(EISGov_st7), prio3/4(EISGov_st7), prio4/4(EISGov_st7), prio5/4(EISGov_st7)
  EISGov_st1/1 -> prio1/1(EISGov_st1), prio2/1(EISGov_st1), prio3/1(EISGov_st1), prio4/1(EISGov_st1), prio5/1(EISGov_st1)
  DrvDem_KpCurrLo_mp/1 -> DrvDem_Parameter/3(DrvDem_KpCurrLo_mp)
  DrvDem_nSetPLo/1 -> DrvDem_Parameter/1(DrvDem_nSetPLo)
  DrvDem_nSetPHi/1 -> DrvDem_Parameter/2(DrvDem_nSetPHi)
  DrvDem_KpPosCurrLo_mp/1 -> DrvDem_Parameter/4(DrvDem_KpPosCurrLo_mp)
  DrvDem_PWinPosLo/1 -> DrvDem_Parameter/6(DrvDem_PWinPosLo)
  DrvDem_KpNegCurrLo_mp/1 -> DrvDem_Parameter/5(DrvDem_KpNegCurrLo_mp)
  DrvDem_PWinNegLo/1 -> DrvDem_Parameter/7(DrvDem_PWinNegLo)
  DrvDem_KiCurrLo_mp/1 -> DrvDem_Parameter/8(DrvDem_KiCurrLo_mp)
  DrvDem_KiPosCurrLo_mp/1 -> DrvDem_Parameter/9(DrvDem_KiPosCurrLo_mp)
  DrvDem_KiNegCurrLo_mp/1 -> DrvDem_Parameter/10(DrvDem_KiNegCurrLo_mp)
  DrvDem_PWinNegHi/1 -> DrvDem_Parameter/17(DrvDem_PWinNegHi)
  DrvDem_KpPosCurrHi_mp/1 -> DrvDem_Parameter/14(DrvDem_KpPosCurrHi_mp)
  DrvDem_IWinNegLo/1 -> DrvDem_Parameter/12(DrvDem_IWinNegLo)
  DrvDem_KpNegCurrHi_mp/1 -> DrvDem_Parameter/15(DrvDem_KpNegCurrHi_mp)
  DrvDem_KiPosCurrHi_mp/1 -> DrvDem_Parameter/19(DrvDem_KiPosCurrHi_mp)
  DrvDem_KiNegCurrHi_mp/1 -> DrvDem_Parameter/20(DrvDem_KiNegCurrHi_mp)
  DrvDem_IWinPosLo/1 -> DrvDem_Parameter/11(DrvDem_IWinPosLo)
  DrvDem_KpCurrHi_mp/1 -> DrvDem_Parameter/13(DrvDem_KpCurrHi_mp)
  DrvDem_IWinNegHi/1 -> DrvDem_Parameter/22(DrvDem_IWinNegHi)
  DrvDem_PWinPosHi/1 -> DrvDem_Parameter/16(DrvDem_PWinPosHi)
  DrvDem_IWinPosHi/1 -> DrvDem_Parameter/21(DrvDem_IWinPosHi)
  DrvDem_KiCurrHi_mp/1 -> DrvDem_Parameter/18(DrvDem_KiCurrHi_mp)
  DrvDem_trqReq/1 -> DrvDem_Parameter/23(DrvDem_trqReq)
  WESDem_KpNegCurrLo_mp/1 -> WESDem_Parameter/6(WESDem_KpNegCurrLo_mp)
  WESDem_KpNegCurrHi_mp/1 -> WESDem_Parameter/5(WESDem_KpNegCurrHi_mp)
  WESDem_PWinNegHi/1 -> WESDem_Parameter/9(WESDem_PWinNegHi)
  WESDem_KpCurrHi_mp/1 -> WESDem_Parameter/1(WESDem_KpCurrHi_mp)
  WESDem_KpCurrLo_mp/1 -> WESDem_Parameter/2(WESDem_KpCurrLo_mp)
  WESDem_PWinPosHi/1 -> WESDem_Parameter/7(WESDem_PWinPosHi)
  WESDem_KpPosCurrHi_mp/1 -> WESDem_Parameter/3(WESDem_KpPosCurrHi_mp)
  WESDem_PWinPosLo/1 -> WESDem_Parameter/8(WESDem_PWinPosLo)
  WESDem_PWinNegLo/1 -> WESDem_Parameter/10(WESDem_PWinNegLo)
  WESDem_KpPosCurrLo_mp/1 -> WESDem_Parameter/4(WESDem_KpPosCurrLo_mp)
  WESDem_nSetPLo/1 -> WESDem_Parameter/22(WESDem_nSetPHi)
  WESDem_IWinNegHi/1 -> WESDem_Parameter/17(WESDem_IWinNegHi)
  WESDem_IWinPosHi/1 -> WESDem_Parameter/19(WESDem_IWinPosHi)
  WESDem_KiCurrLo_mp/1 -> WESDem_Parameter/12(WESDem_KiCurrLo_mp)
  WESDem_KiNegCurrHi_mp/1 -> WESDem_Parameter/13(WESDem_KiNegCurrHi_mp)
  WESDem_nSetPHi/1 -> WESDem_Parameter/23(WESDem_nSetPLo)
  WESDem_IWinPosLo/1 -> WESDem_Parameter/20(WESDem_IWinPosLo)
  WESDem_KiPosCurrHi_mp/1 -> WESDem_Parameter/15(WESDem_KiPosCurrHi_mp)
  WESDem_KiCurrHi_mp/1 -> WESDem_Parameter/11(WESDem_KiCurrHi_mp)
  WESDem_KiPosCurrLo_mp/1 -> WESDem_Parameter/16(WESDem_KiPosCurrLo_mp)
  WESDem_KiNegCurrLo_mp/1 -> WESDem_Parameter/14(WESDem_KiNegCurrLo_mp)
  WESDem_IWinNegLo/1 -> WESDem_Parameter/18(WESDem_IWinNegLo)
  WESDem_trqReq/1 -> WESDem_Parameter/21(WESDem_trqReq)
  ExtDem_nSetPHi/1 -> ExtDem_Parameter/21(ExtDem_nSetPHi)
  ExtDem_nSetPLo/1 -> ExtDem_Parameter/22(ExtDem_nSetPLo)
  ExtDem_trqReq/1 -> ExtDem_Parameter/23(ExtDem_trqReq)
  ExtDem_PWinPosLo/1 -> ExtDem_Parameter/1(ExtDem_PWinPosLo)
  ExtDem_PWinNegLo/1 -> ExtDem_Parameter/2(ExtDem_PWinNegLo)
  ExtDem_IWinPosLo/1 -> ExtDem_Parameter/3(ExtDem_IWinPosLo)
  ExtDem_IWinNegHi/1 -> ExtDem_Parameter/8(ExtDem_IWinNegHi)
  ExtDem_IWinNegLo/1 -> ExtDem_Parameter/4(ExtDem_IWinNegLo)
  ExtDem_IWinPosHi/1 -> ExtDem_Parameter/7(ExtDem_IWinPosHi)
  ExtDem_KpCurrLo_mp/1 -> ExtDem_Parameter/10(ExtDem_KpCurrLo_mp)
  ExtDem_PWinPosHi/1 -> ExtDem_Parameter/5(ExtDem_PWinPosHi)
  ExtDem_PWinNegHi/1 -> ExtDem_Parameter/6(ExtDem_PWinNegHi)
  ExtDem_KpPosCurrLo_mp/1 -> ExtDem_Parameter/14(ExtDem_KpPosCurrLo_mp)
  ExtDem_KpNegCurrLo_mp/1 -> ExtDem_Parameter/12(ExtDem_KpNegCurrLo_mp)
  ExtDem_KiCurrHi_mp/1 -> ExtDem_Parameter/15(ExtDem_KiCurrHi_mp)
  ExtDem_KiCurrLo_mp/1 -> ExtDem_Parameter/16(ExtDem_KiCurrLo_mp)
  ExtDem_KiPosCurrLo_mp/1 -> ExtDem_Parameter/20(ExtDem_KiPosCurrLo_mp)
  ExtDem_KpNegCurrHi_mp/1 -> ExtDem_Parameter/11(ExtDem_KpNegCurrHi_mp)
  ExtDem_KpCurrHi_mp/1 -> ExtDem_Parameter/9(ExtDem_KpCurrHi_mp)
  ExtDem_KpPosCurrHi_mp/1 -> ExtDem_Parameter/13(ExtDem_KpPosCurrHi_mp)
  ExtDem_KiNegCurrHi_mp/1 -> ExtDem_Parameter/17(ExtDem_KiNegCurrHi_mp)
  ExtDem_KiNegCurrLo_mp/1 -> ExtDem_Parameter/18(ExtDem_KiNegCurrLo_mp)
  ExtDem_KiPosCurrHi_mp/1 -> ExtDem_Parameter/19(ExtDem_KiPosCurrHi_mp)
  Relational Operator8/1 -> Switch5/2
  Relational Operator6/1 -> Switch6/2
  Relational Operator7/1 -> Switch7/2
  Relational Operator5/1 -> Switch8/2
  Switch5/1 -> Switch6/3
  Switch6/1 -> Switch7/3
  Switch7/1 -> Switch8/3
  Delay1/1 -> Switch5/3
  Constant/1 -> Relational Operator9/1, Switch5/1
  Constant13/1 -> Relational Operator10/1, Switch6/1
  Relational Operator9/1 -> HLSDem_Parameter/Enable
  Relational Operator10/1 -> DrvDem_Parameter/Enable
  Constant14/1 -> Relational Operator11/1, Switch7/1
  Relational Operator11/1 -> WESDem_Parameter/Enable
  Switch8/1 -> Relational Operator11/2, Relational Operator10/2, Delay1/1, Relational Operator9/2, Relational Operator12/2
  Constant16/1 -> Relational Operator12/1, Switch8/1
  Relational Operator12/1 -> ExtDem_Parameter/Enable
  [HLSDem_nSetPHi] -> EISGov_Parameter/27(HLSDem_nSetPHi_IN)
  Epm_nEng/1 -> EISGov_Parameter/26(Epm_nEng)
  T15_st/1 -> EISGov_Parameter/28(T15_st)

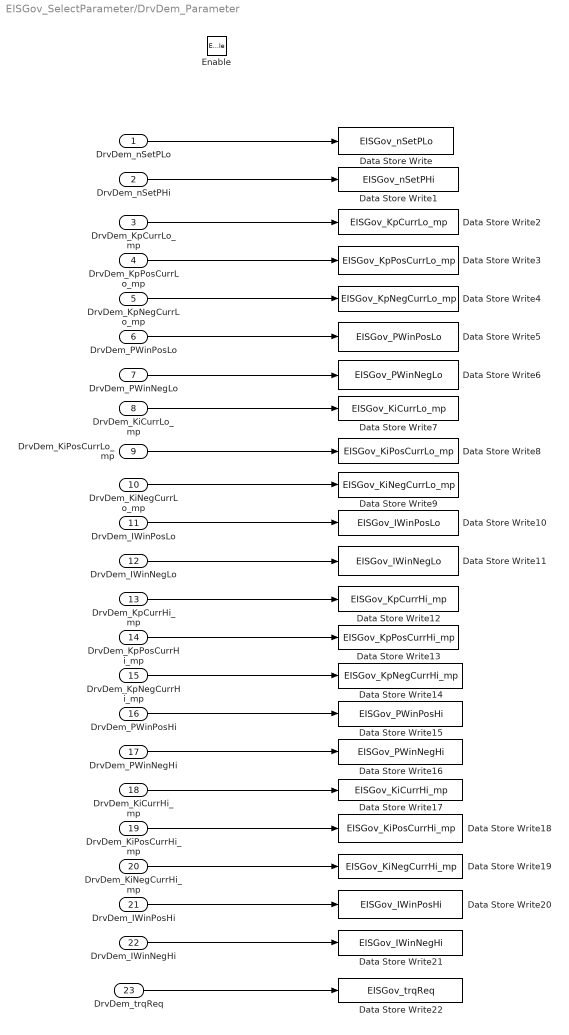
== system EISGov_SelectParameter/DrvDem_Parameter ==
  DrvDem_nSetPLo : Inport
  DrvDem_nSetPHi : Inport  Port=2
  DrvDem_KpCurrLo_mp : Inport  Port=3
  DrvDem_KpPosCurrLo_mp : Inport  Port=4
  DrvDem_KpNegCurrLo_mp : Inport  Port=5
  DrvDem_PWinPosLo : Inport  Port=6
  DrvDem_PWinNegLo : Inport  Port=7
  DrvDem_KiCurrLo_mp : Inport  Port=8
  DrvDem_KiPosCurrLo_mp : Inport  Port=9
  DrvDem_KiNegCurrLo_mp : Inport  Port=10
  DrvDem_IWinPosLo : Inport  Port=11
  DrvDem_IWinNegLo : Inport  Port=12
  DrvDem_KpCurrHi_mp : Inport  Port=13
  DrvDem_KpPosCurrHi_mp : Inport  Port=14
  DrvDem_KpNegCurrHi_mp : Inport  Port=15
  DrvDem_PWinPosHi : Inport  Port=16
  DrvDem_PWinNegHi : Inport  Port=17
  DrvDem_KiCurrHi_mp : Inport  Port=18
  DrvDem_KiPosCurrHi_mp : Inport  Port=19
  DrvDem_KiNegCurrHi_mp : Inport  Port=20
  DrvDem_IWinPosHi : Inport  Port=21
  DrvDem_IWinNegHi : Inport  Port=22
  DrvDem_trqReq : Inport  Port=23
  Enable : EnablePort
  Data Store Write : DataStoreWrite  DataStoreName=EISGov_nSetPLo
  Data Store Write1 : DataStoreWrite  DataStoreName=EISGov_nSetPHi
  Data Store Write10 : DataStoreWrite  DataStoreName=EISGov_IWinPosLo
  Data Store Write11 : DataStoreWrite  DataStoreName=EISGov_IWinNegLo
  Data Store Write12 : DataStoreWrite  DataStoreName=EISGov_KpCurrHi_mp
  Data Store Write13 : DataStoreWrite  DataStoreName=EISGov_KpPosCurrHi_mp
  Data Store Write14 : DataStoreWrite  DataStoreName=EISGov_KpNegCurrHi_mp
  Data Store Write15 : DataStoreWrite  DataStoreName=EISGov_PWinPosHi
  Data Store Write16 : DataStoreWrite  DataStoreName=EISGov_PWinNegHi
  Data Store Write17 : DataStoreWrite  DataStoreName=EISGov_KiCurrHi_mp
  Data Store Write18 : DataStoreWrite  DataStoreName=EISGov_KiPosCurrHi_mp
  Data Store Write19 : DataStoreWrite  DataStoreName=EISGov_KiNegCurrHi_mp
  Data Store Write2 : DataStoreWrite  DataStoreName=EISGov_KpCurrLo_mp
  Data Store Write20 : DataStoreWrite  DataStoreName=EISGov_IWinPosHi
  Data Store Write21 : DataStoreWrite  DataStoreName=EISGov_IWinNegHi
  Data Store Write22 : DataStoreWrite  DataStoreName=EISGov_trqReq
  Data Store Write3 : DataStoreWrite  DataStoreName=EISGov_KpPosCurrLo_mp
  Data Store Write4 : DataStoreWrite  DataStoreName=EISGov_KpNegCurrLo_mp
  Data Store Write5 : DataStoreWrite  DataStoreName=EISGov_PWinPosLo
  Data Store Write6 : DataStoreWrite  DataStoreName=EISGov_PWinNegLo
  Data Store Write7 : DataStoreWrite  DataStoreName=EISGov_KiCurrLo_mp
  Data Store Write8 : DataStoreWrite  DataStoreName=EISGov_KiPosCurrLo_mp
  Data Store Write9 : DataStoreWrite  DataStoreName=EISGov_KiNegCurrLo_mp
  wires:
  DrvDem_PWinPosLo/1 -> Data Store Write5/1
  DrvDem_PWinNegLo/1 -> Data Store Write6/1
  DrvDem_KiCurrLo_mp/1 -> Data Store Write7/1
  DrvDem_KiPosCurrLo_mp/1 -> Data Store Write8/1
  DrvDem_KiNegCurrLo_mp/1 -> Data Store Write9/1
  DrvDem_IWinPosLo/1 -> Data Store Write10/1
  DrvDem_IWinNegLo/1 -> Data Store Write11/1
  DrvDem_KpCurrHi_mp/1 -> Data Store Write12/1
  DrvDem_KpPosCurrHi_mp/1 -> Data Store Write13/1
  DrvDem_KpNegCurrHi_mp/1 -> Data Store Write14/1
  DrvDem_PWinPosHi/1 -> Data Store Write15/1
  DrvDem_PWinNegHi/1 -> Data Store Write16/1
  DrvDem_KiCurrHi_mp/1 -> Data Store Write17/1
  DrvDem_KiPosCurrHi_mp/1 -> Data Store Write18/1
  DrvDem_KiNegCurrHi_mp/1 -> Data Store Write19/1
  DrvDem_IWinPosHi/1 -> Data Store Write20/1
  DrvDem_IWinNegHi/1 -> Data Store Write21/1
  DrvDem_nSetPLo/1 -> Data Store Write/1
  DrvDem_nSetPHi/1 -> Data Store Write1/1
  DrvDem_KpCurrLo_mp/1 -> Data Store Write2/1
  DrvDem_KpPosCurrLo_mp/1 -> Data Store Write3/1
  DrvDem_KpNegCurrLo_mp/1 -> Data Store Write4/1
  DrvDem_trqReq/1 -> Data Store Write22/1
